simulink model "CaseDemuxThree"  (R2023b)
settings: Solver=VariableStepAuto  StartTime=0.0  StopTime=10.0  RelTol=1e-3
settings Model: Creator=jsonm  LastModifiedBy=jsonm

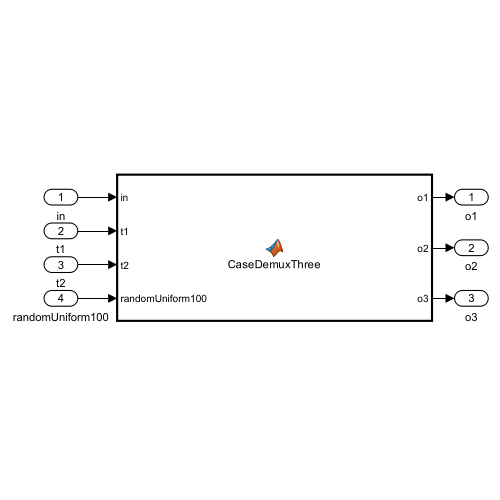
[thumbnail: Simulink's stored preview of the top-level diagram]
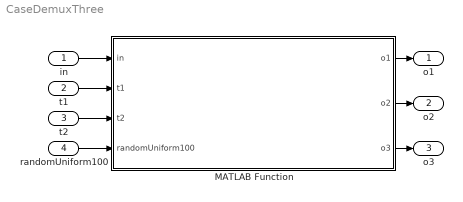
== system CaseDemuxThree ==
  in : Inport
  t1 : Inport  Port=2
  t2 : Inport  Port=3
  randomUniform100 : Inport  Port=4
  MATLAB Function : MATLAB Function  TreatAsAtomicUnit=on
  o1 : Outport
  o2 : Outport  Port=2
  o3 : Outport  Port=3
  wires:
  MATLAB Function/1(o1) -> o1/1
  MATLAB Function/2(o2) -> o2/1
  in/1 -> MATLAB Function/1(in)
  t1/1 -> MATLAB Function/2(t1)
  t2/1 -> MATLAB Function/3(t2)
  MATLAB Function/3(o3) -> o3/1
  randomUniform100/1 -> MATLAB Function/4(randomUniform100)

== matlab function CaseDemuxThree/MATLAB Function ==
  data: in input; o1 output; t1 input; o2 output; t2 input; o3 output; randomUniform100 input
function [o1, o2, o3] = CaseDemuxThree(in, t1, t2, randomUniform100)

% Method to demux input into one of three possible outputs based on
% probabilities.
%
% t1 is a threshold bound between 0 and 100 used as follows
% x = rand*100
% 0 <= x < t1 => o1
%
% Negative is a non-valid output
%
% Written by Darian Muresan
% Modified by Jason McCauley

o1 = -1;
o2 = -1;
o3 = -1;

if nargin < 4
    x = rand*100; % If randomUniform100 is not provided, generate a random number
else
    x = randomUniform100; % randomUniform100 uses different seeds to generate random number, use if provided at each CaseDemux
end

if (0 <= x && x <= t1)
    o1 = in;
elseif (t1 < x && x <= t2)
    o2 = in;
else
    o3 = in;
end
